simulink model "KalmanFilter"  (R2016a)
settings: Solver=VariableStepAuto  StartTime=0.0  StopTime=10.0  RelTol=1e-3
values from neighbouring files (symbols this model uses):
  A = [1.00008442099 -8.64762700945e-06 -0.00202879786618 -0.0120769175733 -0.00073933561133 1.00039660277 -0.00870367805975 0.00595527209343 -0.00126263380998 0.00387872249587 0.98705447221 -0.0360153373111 ... (16 elements, 4x4)]    [sample.mat]
  B = [-5.50080453987e-08  3.86684801471e-08; 8.77127889262e-08  -5.25096440473e-08; 1.59329018214e-07  1.46974501157e-09; -2.9421226826e-06  9.98312400046e-06]    [sample.mat]
  C = Cbar*C_new    [Params.m]    (also in sample.mat = [0.219326280868  0.071395429974  0.0140743658612  0.00013653)
  P00 = [1 1 1 1 1 1 1 1 1 1 1 1 ... (16 elements, 4x4)]    [sample.mat]
  Q = [1 0 0 0 0 1 0 0 0 0 1 0 ... (16 elements, 4x4)]    [sample.mat]
  R = 8.3143e-3    (= 0.0083143)    [Yrates.m]    (also in sample.mat = [0.01  0  0; 0  0.01  0; 0  0  0.01])
  u0 = [1 1]    [sample.mat]
  X00 = [0.0472364555772 -0.0576472307603 -0.165494284832 -0.106452387138]    [sample.mat]
  Ymeas = Cin(N*p+1:N*p+N)    [Controller.m]    (also in sample.mat = [2 2 200])
settings Model: Creator=hp  LastModifiedBy=hp

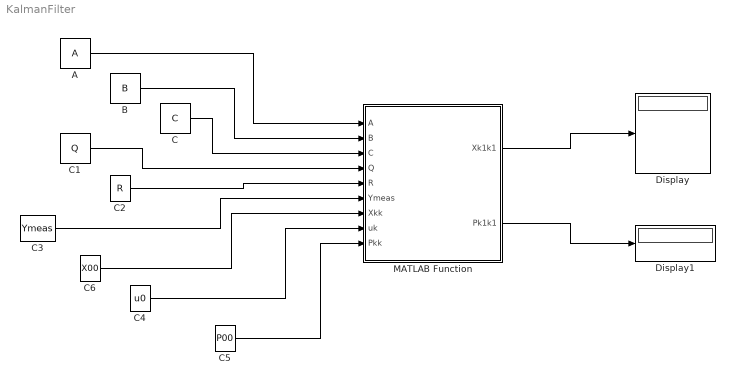
== system KalmanFilter ==
  A : Constant  Value=A  VectorParams1D=off
  B : Constant  Value=B  VectorParams1D=off
  C : Constant  Value=C  VectorParams1D=off
  C1 : Constant  Value=Q  VectorParams1D=off
  C2 : Constant  Value=R  VectorParams1D=off
  C3 : Constant  Value=Ymeas  VectorParams1D=off
  C4 : Constant  Value=u0  VectorParams1D=off
  C5 : Constant  Value=P00  VectorParams1D=off
  C6 : Constant  Value=X00  VectorParams1D=off
  Display : Display
  Display1 : Display
  MATLAB Function : MATLAB Function  TreatAsAtomicUnit=on
  wires:
  A/1 -> MATLAB Function/1(A)
  B/1 -> MATLAB Function/2(B)
  C/1 -> MATLAB Function/3(C)
  C1/1 -> MATLAB Function/4(Q)
  C2/1 -> MATLAB Function/5(R)
  C3/1 -> MATLAB Function/6(Ymeas)
  C4/1 -> MATLAB Function/8(uk)
  C5/1 -> MATLAB Function/9(Pkk)
  C6/1 -> MATLAB Function/7(Xkk)
  MATLAB Function/1(Xk1k1) -> Display/1
  MATLAB Function/2(Pk1k1) -> Display1/1

== matlab function KalmanFilter/MATLAB Function ==
  data: A input; Xk1k1 output; B input; C input; Q input; R input; Ymeas input; Xkk input; uk input; Pkk input; Pk1k1 output
function [Xk1k1,Pk1k1] = KalmanFilter(A,B,C,Q,R,Ymeas,Xkk,uk,Pkk)


s     = size(Pkk);
    % Prediction
    Xk1k=A*Xkk+B*uk;
    Pk1k=A*Pkk*A'+Q;
     % Correction
    K=Pk1k*C'*inv(C*Pk1k*C'+R);        % Optimal Kalman gain
    Xk1k1=Xk1k+K*(Ymeas-C*Xk1k);
    
    Pk1k1=(eye(s)-K*C)*Pk1k;


end
